simulink model "Model"  (R2012b)
settings: Solver=ode45  StartTime=0.0  StopTime=2000  RelTol=1e-3
values from neighbouring files (symbols this model uses):
  Kt = 1    [Coeff.m]
  Kv = 0.05    [Coeff.m]
  L = 2    [Coeff.m]
  x_final = 400    [Coeff.m]
  y_final = 200    [Coeff.m]
libraries: simulink x3
settings Model: Creator=kuparez  LastModifiedBy=kuparez

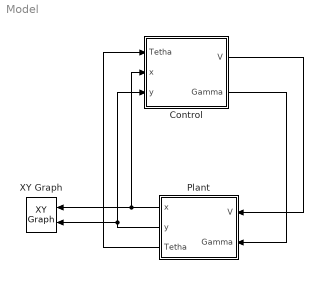
== system Model ==
  Control : Subsystem
  Plant : Subsystem
  XY Graph : simulink/Sinks/XY Graph  xmin=0  xmax=500  ymin=0  ymax=500  st=-1
  wires:
  Control/1(V) -> Plant/1(V)
  Control/2(Gamma) -> Plant/2(Gamma)
  Plant/1(x) -> XY Graph/1, Control/2(x)
  Plant/2(y) -> XY Graph/2, Control/3(y)
  Plant/3(Tetha) -> Control/1(Tetha)

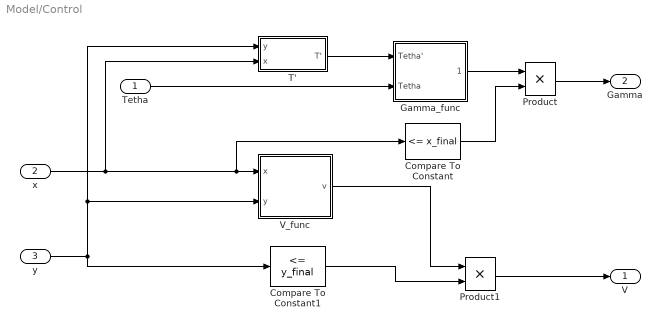
== system Model/Control ==
  Tetha : Inport
  x : Inport  Port=2
  y : Inport  Port=3
  Compare To Constant : simulink/Logic and Bit Operations/Compare To Constant  relop=<=  const=x_final  OutDataTypeStr=boolean
  Compare To Constant1 : simulink/Logic and Bit Operations/Compare To Constant  relop=<=  const=y_final  OutDataTypeStr=boolean
  Gamma_func : Subsystem
  Product : Product  RndMeth=Zero
  Product1 : Product  RndMeth=Zero
  T' : Subsystem
  V_func : Subsystem
  V : Outport
  Gamma : Outport  Port=2
  wires:
  T'/1(T') -> Gamma_func/1(Tetha')
  Tetha/1 -> Gamma_func/2(Tetha)
  x/1 -> Compare To Constant/1, V_func/1(x), T'/2(x)
  y/1 -> Compare To Constant1/1, T'/1(y), V_func/2(y)
  Gamma_func/1(Gamma) -> Product/1
  Product/1 -> Gamma/1
  Compare To Constant/1 -> Product/2
  Product1/1 -> V/1
  Compare To Constant1/1 -> Product1/2
  V_func/1(v) -> Product1/1

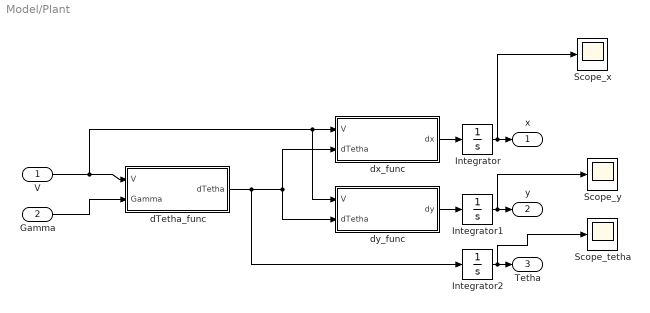
== system Model/Plant ==
  V : Inport
  Gamma : Inport  Port=2
  Integrator : Integrator
  Integrator1 : Integrator
  Integrator2 : Integrator
  Scope_tetha : Scope
      settings: YMin=0  YMax=22.5  SaveName=ScopeData4
  Scope_x : Scope
      settings: YMin=0  YMax=400  SaveName=ScopeData2
  Scope_y : Scope
      settings: YMin=0  YMax=250  SaveName=ScopeData3
  dTetha_func : Subsystem
  dx_func : Subsystem
  dy_func : Subsystem
  x : Outport
  y : Outport  Port=2
  Tetha : Outport  Port=3
  wires:
  Gamma/1 -> dTetha_func/2(Gamma)
  V/1 -> dy_func/1(V), dx_func/1(V), dTetha_func/1(V)
  dy_func/1(dy) -> Integrator1/1
  dx_func/1(dx) -> Integrator/1
  Integrator1/1 -> Scope_y/1, y/1
  dTetha_func/1(dTetha) -> Integrator2/1, dy_func/2(dTetha), dx_func/2(dTetha)
  Integrator2/1 -> Scope_tetha/1, Tetha/1
  Integrator/1 -> Scope_x/1, x/1

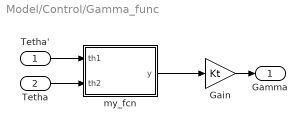
== system Model/Control/Gamma_func ==
  Tetha' : Inport
  Tetha : Inport  Port=2
  Gain : Gain  Gain=Kt
  my_fcn : MATLAB Function  TreatAsAtomicUnit=on
  Gamma : Outport
  wires:
  my_fcn/1(y) -> Gain/1
  Tetha'/1 -> my_fcn/1(th1)
  Gain/1 -> Gamma/1
  Tetha/1 -> my_fcn/2(th2)

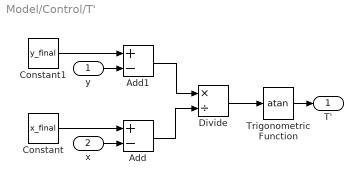
== system Model/Control/T' ==
  y : Inport
  x : Inport  Port=2
  Add : Sum  Inputs=+-
  Add1 : Sum  Inputs=+-
  Constant : Constant  Value=x_final
  Constant1 : Constant  Value=y_final
  Divide : Product  Inputs=*/
  Trigonometric Function : Trigonometry  Operator=atan
  T' : Outport
  wires:
  Trigonometric Function/1 -> T'/1
  Constant/1 -> Add/1
  Add1/1 -> Divide/1
  Add/1 -> Divide/2
  x/1 -> Add/2
  y/1 -> Add1/2
  Divide/1 -> Trigonometric Function/1
  Constant1/1 -> Add1/1

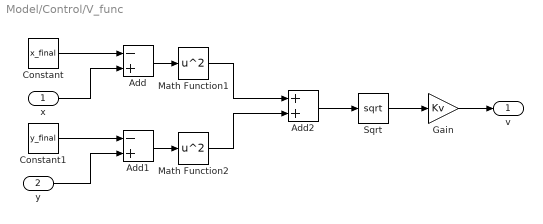
== system Model/Control/V_func ==
  x : Inport
  y : Inport  Port=2
  Add : Sum  Inputs=-+
  Add1 : Sum  Inputs=-+
  Add2 : Sum
  Constant : Constant  Value=x_final
  Constant1 : Constant  Value=y_final
  Gain : Gain  Gain=Kv
  Math Function1 : Math  Operator=square  SaturateOnIntegerOverflow=on
  Math Function2 : Math  Operator=square  SaturateOnIntegerOverflow=on
  Sqrt : Sqrt  SaturateOnIntegerOverflow=on
  v : Outport
  wires:
  y/1 -> Add1/2
  Add1/1 -> Math Function2/1
  Add/1 -> Math Function1/1
  x/1 -> Add/2
  Constant/1 -> Add/1
  Math Function2/1 -> Add2/2
  Add2/1 -> Sqrt/1
  Constant1/1 -> Add1/1
  Math Function1/1 -> Add2/1
  Gain/1 -> v/1
  Sqrt/1 -> Gain/1

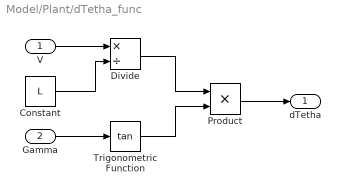
== system Model/Plant/dTetha_func ==
  V : Inport
  Gamma : Inport  Port=2
  Constant : Constant  Value=L
  Divide : Product  Inputs=*/
  Product : Product  RndMeth=Zero
  Trigonometric Function : Trigonometry  Operator=tan
  dTetha : Outport
  wires:
  Constant/1 -> Divide/2
  V/1 -> Divide/1
  Gamma/1 -> Trigonometric Function/1
  Trigonometric Function/1 -> Product/2
  Divide/1 -> Product/1
  Product/1 -> dTetha/1

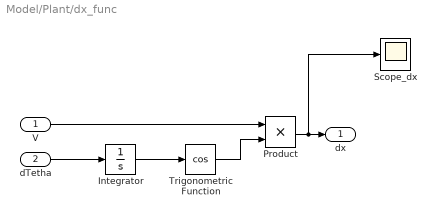
== system Model/Plant/dx_func ==
  V : Inport
  dTetha : Inport  Port=2
  Integrator : Integrator
  Product : Product  RndMeth=Zero
  Scope_dx : Scope
      settings: YMin=-150  YMax=400
  Trigonometric Function : Trigonometry  Operator=cos
  dx : Outport
  wires:
  dTetha/1 -> Integrator/1
  Integrator/1 -> Trigonometric Function/1
  Trigonometric Function/1 -> Product/2
  V/1 -> Product/1
  Product/1 -> Scope_dx/1, dx/1

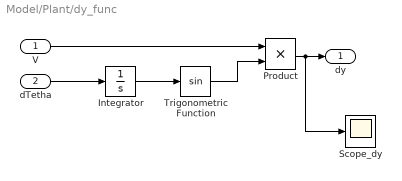
== system Model/Plant/dy_func ==
  V : Inport
  dTetha : Inport  Port=2
  Integrator : Integrator
  Product : Product  RndMeth=Zero
  Scope_dy : Scope
      settings: YMin=-250  YMax=1750
  Trigonometric Function : Trigonometry
  dy : Outport
  wires:
  dTetha/1 -> Integrator/1
  Integrator/1 -> Trigonometric Function/1
  Trigonometric Function/1 -> Product/2
  V/1 -> Product/1
  Product/1 -> Scope_dy/1, dy/1

== matlab function Model/Control/Gamma_func/my_fcn ==
  data: th1 input; y output; th2 input
function y = my_fcn(th1, th2)
%#codegen

    if nargin < 2
        d = th1;
    else
        d = th1 - th2;
    end
    d = mod(d+pi, 2*pi) - pi;
y = d;
